simulink model "ZLShPID"  (Simulink 5.0)
settings: Solver=ode45  StartTime=0.0  StopTime=1.0  RelTol=1e-3
settings Model: LastModifiedBy=ThinkPad

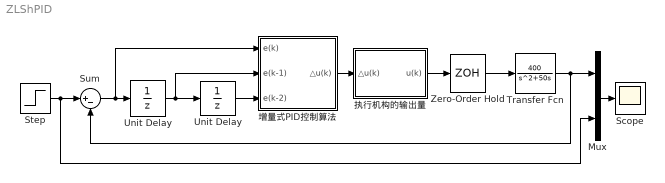
== system ZLShPID ==
  Mux : Mux  Inputs=2
  Scope : Scope
      settings: YMin=0  YMax=1.25  SaveName=ZLShPID  DataFormat=Array  MaxDataPoints=50000
  Step : Step  Time=0  SampleTime=0
  Sum : Sum  Inputs=|+-  SaturateOnIntegerOverflow=on
  Transfer Fcn : TransferFcn  Numerator=[400]  Denominator=[1 50 0]
  Unit Delay : UnitDelay  SampleTime=0.001
  "Unit Delay " : UnitDelay  SampleTime=0.001
  "Zero-Order Hold " : ZeroOrderHold  SampleTime=0.001
  增量式PID控制算法 : Subsystem
  执行机构的输出量 : Subsystem
  wires:
  Step/1 -> Sum/1, Mux/2
  Sum/1 -> 增量式PID控制算法/1(e(k)), Unit Delay/1
  Mux/1 -> Scope/1
  Transfer Fcn/1 -> Sum/2, Mux/1
  Unit Delay/1 -> 增量式PID控制算法/2(e(k-1)), "Unit Delay "/1
  "Unit Delay "/1 -> 增量式PID控制算法/3(e(k-2))
  "Zero-Order Hold "/1 -> Transfer Fcn/1
  增量式PID控制算法/1("△u(k) ") -> 执行机构的输出量/1("△u(k) ")
  执行机构的输出量/1(u(k)) -> "Zero-Order Hold "/1

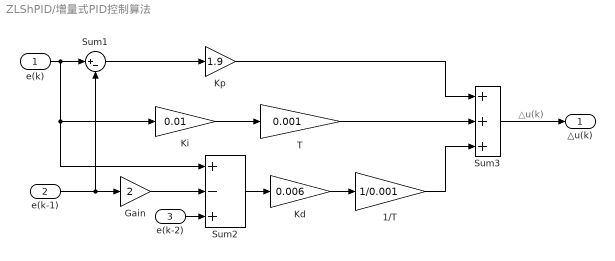
== system ZLShPID/增量式PID控制算法 ==
  note: △u(k)
  e(k) : Inport
  e(k-1) : Inport  Port=2
  e(k-2) : Inport  Port=3
  1/T : Gain  Gain=1/0.001  SaturateOnIntegerOverflow=on
  Gain : Gain  Gain=2  SaturateOnIntegerOverflow=on
  Kd : Gain  Gain=0.006  SaturateOnIntegerOverflow=on
  Ki : Gain  Gain=0.01  SaturateOnIntegerOverflow=on
  Kp : Gain  Gain=1.9  SaturateOnIntegerOverflow=on
  Sum1 : Sum  Inputs=|+-  SaturateOnIntegerOverflow=on
  Sum2 : Sum  Inputs=+-+  SaturateOnIntegerOverflow=on
  Sum3 : Sum  Inputs=+++  SaturateOnIntegerOverflow=on
  T : Gain  Gain=0.001  SaturateOnIntegerOverflow=on
  "△u(k) " : Outport
  wires:
  Sum1/1 -> Kp/1
  Gain/1 -> Sum2/2
  Sum2/1 -> Kd/1
  e(k-1)/1 -> Gain/1, Sum1/2
  e(k-2)/1 -> Sum2/3
  e(k)/1 -> Sum1/1, Sum2/1, Ki/1
  Kp/1 -> Sum3/1
  Ki/1 -> T/1
  Sum3/1 -> "△u(k) "/1
  Kd/1 -> 1/T/1
  T/1 -> Sum3/2
  1/T/1 -> Sum3/3

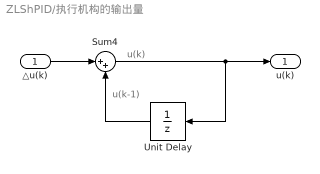
== system ZLShPID/执行机构的输出量 ==
  note: u(k-1)
  note: u(k)
  "△u(k) " : Inport
  Sum4 : Sum  Inputs=|++  SaturateOnIntegerOverflow=on
  Unit Delay : UnitDelay  Orientation=left  SampleTime=0.001
  u(k) : Outport
  wires:
  Sum4/1 -> Unit Delay/1, u(k)/1
  Unit Delay/1 -> Sum4/2
  "△u(k) "/1 -> Sum4/1
